simulink model "Project2_1a_AbhayKela"  (R2014b)
settings: Solver=ode5  StartTime=0.0  StopTime=tf  FixedStep=0.01  RelTol=1e-3
values from neighbouring files (symbols this model uses):
  x1 = xm    (= 0)    [HW2_Bisection_f_AbhayKela.m]    (also in HW2_Bisection_x_AbhayKela.m; HW2_Cubicsearch_f_AbhayKela.m = xm; HW2_Cubicsearch_x_AbhayKela.m = xm; HW2_Goldensection_AbhayKela.m = 1.11456139059)
  x2 = xm    (= 0)    [HW2_Bisection_f_AbhayKela.m]    (also in HW2_Bisection_x_AbhayKela.m; HW2_Cubicsearch_f_AbhayKela.m = 20; HW2_Cubicsearch_x_AbhayKela.m = 20; HW2_Goldensection_AbhayKela.m = 4.72136)
settings Model: Creator=axk7578  LastModifiedBy=axk7578

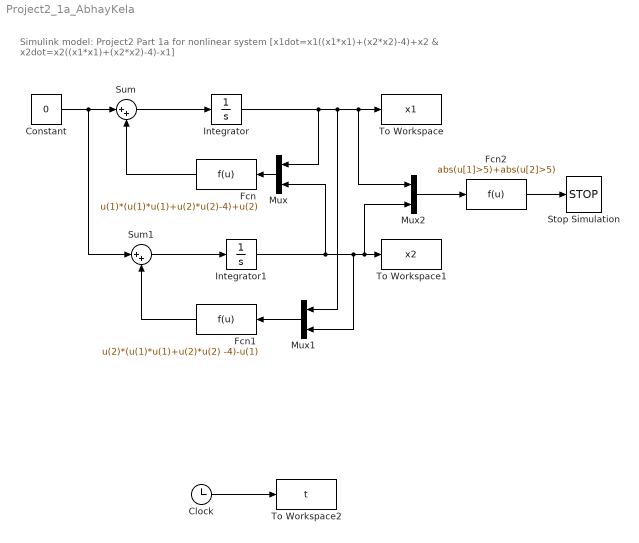
== system Project2_1a_AbhayKela ==
  note: Simulink model: Project2 Part 1a for nonlinear system [x1dot=x1((x1*x1)+(x2*x2)-4)+x2 & x2dot=x2((x1*x1)+(x2*x2)-4)-x1]
  Clock : Clock
  Constant : Constant  Value=0
  Fcn : Fcn  Expr=u(1)*(u(1)*u(1)+u(2)*u(2)-4)+u(2)
  Fcn1 : Fcn  Expr=u(2)*(u(1)*u(1)+u(2)*u(2) -4)-u(1)
  Fcn2 : Fcn  Expr=abs(u[1]>5)+abs(u[2]>5)
  Integrator : Integrator  InitialCondition=x1
  Integrator1 : Integrator  InitialCondition=x2
  Mux : Mux  Inputs=2
  Mux1 : Mux  Inputs=2
  Mux2 : Mux  Inputs=2
  Stop Simulation : Stop
  Sum : Sum  Inputs=|++
  Sum1 : Sum  Inputs=|++
  To Workspace : ToWorkspace  VariableName=x1  SampleTime=-1
  To Workspace1 : ToWorkspace  VariableName=x2  SampleTime=-1
  To Workspace2 : ToWorkspace  VariableName=t  SampleTime=-1
  wires:
  Sum/1 -> Integrator/1
  Sum1/1 -> Integrator1/1
  Fcn/1 -> Sum/2
  Mux/1 -> Fcn/1
  Integrator1/1 -> Mux1/2, Mux2/2, To Workspace1/1, Mux/2
  Integrator/1 -> Mux/1, Mux1/1, Mux2/1, To Workspace/1
  Fcn1/1 -> Sum1/2
  Mux1/1 -> Fcn1/1
  Clock/1 -> To Workspace2/1
  Mux2/1 -> Fcn2/1
  Fcn2/1 -> Stop Simulation/1
  Constant/1 -> Sum1/1, Sum/1
